simulink library "mylib"  (R2020a)
settings: Solver=VariableStepAuto  StartTime=0.0  StopTime=10.0  RelTol=1e-3
undefined symbols (not defined in the file): d_du_max_pu, dir_to_bus1, dir_to_bus_0L, dir_to_bus_2, dir_to_line1, dir_to_line_0L, dir_to_line_2, du_max_pu, du_ph_max_pu, Fi_0, Fi_T_H, Fi_T_L, Fi_T_M, I0_calc_0L, I0_comp_H, I0_comp_L, I0_comp_M, I0_max_0L, I2_max_2, I_diff1, I_diff2, I_diff3, I_diff4, I_diff5, I_diff_to, I_hight_CT1_G, I_hight_CT2_G, I_low_CT1, I_low_CT2, I_max1, I_max2, I_max3, I_max4, I_max5, I_min_sec_CT1, I_min_sec_CT2, I_unb, Iph_max_0L, Iph_max_2, jmp_in_zone, jmp_in_zone_0L, jmp_in_zone_2, K_dop, max_min1, only_K1_0L, only_K1_2, only_K2_0L, only_K2_2, only_K3_0L, only_K3_2, P_ctl_0, PQ_Fi_ctl_0, Q_ctl_0, S_set_0, set, set1, T_fast, T_I_ctl, T_off, T_on ... (+15)
libraries: $bdroot x184, powerlib_meascontrol x97
(part 8 of 14)

== system mylib/Inverse time-delay/ANSI Inverse time-delay/Сoefficient_6 ==
  A_in : Inport
  B_in : Inport  Port=2
  C_in : Inport  Port=3
  N : Inport  Port=4
  Constant1 : Constant  Value=0.02434
  Constant3 : Constant  Value=2
  Constant6 : Constant  Value=5.64
  Switch : Switch  Criteria=u2 > Threshold
  Switch1 : Switch  Criteria=u2 > Threshold
  Switch2 : Switch  Criteria=u2 > Threshold
  A_out : Outport
  B_out : Outport  Port=2
  C_out : Outport  Port=3
  wires:
  Switch1/1 -> B_out/1
  Constant3/1 -> Switch/1
  Constant6/1 -> Switch1/1
  Switch/1 -> A_out/1
  N/1 -> Switch2/2, Switch/2, Switch1/2
  A_in/1 -> Switch/3
  B_in/1 -> Switch1/3
  C_in/1 -> Switch2/3
  Constant1/1 -> Switch2/1
  Switch2/1 -> C_out/1

== system mylib/Inverse time-delay/ANSI Inverse time-delay/Сoefficient_7 ==
  A_in : Inport
  B_in : Inport  Port=2
  C_in : Inport  Port=3
  N : Inport  Port=4
  Constant1 : Constant  Value=0.21359
  Constant3 : Constant  Value=1.5825
  Constant6 : Constant  Value=0.4797
  Switch : Switch  Criteria=u2 > Threshold
  Switch1 : Switch  Criteria=u2 > Threshold
  Switch2 : Switch  Criteria=u2 > Threshold
  A_out : Outport
  B_out : Outport  Port=2
  C_out : Outport  Port=3
  wires:
  Switch1/1 -> B_out/1
  Constant3/1 -> Switch/1
  Constant6/1 -> Switch1/1
  Switch/1 -> A_out/1
  N/1 -> Switch2/2, Switch/2, Switch1/2
  A_in/1 -> Switch/3
  B_in/1 -> Switch1/3
  C_in/1 -> Switch2/3
  Constant1/1 -> Switch2/1
  Switch2/1 -> C_out/1

== system mylib/Inverse time-delay/ANSI Inverse time-delay/Сoefficient_8 User ==
  A_in : Inport
  B_in : Inport  Port=2
  C_in : Inport  Port=3
  N : Inport  Port=4
  Au : Inport  Port=5
  Bu : Inport  Port=6
  Cu : Inport  Port=7
  Switch : Switch  Criteria=u2 > Threshold
  Switch1 : Switch  Criteria=u2 > Threshold
  Switch2 : Switch  Criteria=u2 > Threshold
  B_out : Outport
  A_out : Outport  Port=2
  C_out : Outport  Port=3
  wires:
  Switch1/1 -> B_out/1
  Au/1 -> Switch/1
  Bu/1 -> Switch1/1
  Switch/1 -> A_out/1
  N/1 -> Switch2/2, Switch/2, Switch1/2
  A_in/1 -> Switch/3
  B_in/1 -> Switch1/3
  C_in/1 -> Switch2/3
  Cu/1 -> Switch2/1
  Switch2/1 -> C_out/1

== system mylib/Inverse time-delay/ANSI Inverse time-delay inductive disk relay/Equation ANSI_idr ==
  B : Inport
  I : Inport  Port=2
  Ip : Inport  Port=3
  A : Inport  Port=4
  C : Inport  Port=5
  D : Inport  Port=6
  Add : Sum  Inputs=+-
  Add1 : Sum
  Constant3 : Constant
  Divide : Product  Inputs=*/
  Divide1 : Product  Inputs=*/
  Divide3 : Product  Inputs=**
  Math Function : Math  Operator=pow  SaturateOnIntegerOverflow=on
  Zero_check : Subsystem
  Zero_check1 : Subsystem
  td : Outport
  wires:
  I/1 -> Divide/1
  B/1 -> Divide1/1
  D/1 -> Divide3/2
  Divide3/1 -> td/1
  Divide/1 -> Math Function/1
  A/1 -> Math Function/2
  Ip/1 -> Zero_check/1(in)
  Zero_check/1(out) -> Divide/2
  Add/1 -> Zero_check1/1(in)
  Zero_check1/1(out) -> Divide1/2
  Constant3/1 -> Add/1
  Divide1/1 -> Add1/1
  Add1/1 -> Divide3/1
  C/1 -> Add1/2
  Math Function/1 -> Add/2

== system mylib/Inverse time-delay/ANSI Inverse time-delay inductive disk relay/Сoefficient_1 ==
  A_in : Inport
  B_in : Inport  Port=2
  C_in : Inport  Port=3
  N : Inport  Port=4
  Constant1 : Constant  Value=0
  Constant3 : Constant  Value=2.0938
  Constant6 : Constant  Value=8.8
  Switch : Switch  Criteria=u2 > Threshold
  Switch1 : Switch  Criteria=u2 > Threshold
  Switch2 : Switch  Criteria=u2 > Threshold
  A_out : Outport
  B_out : Outport  Port=2
  C_out : Outport  Port=3
  wires:
  Switch1/1 -> B_out/1
  Constant3/1 -> Switch/1
  Constant6/1 -> Switch1/1
  Switch/1 -> A_out/1
  N/1 -> Switch2/2, Switch/2, Switch1/2
  A_in/1 -> Switch/3
  B_in/1 -> Switch1/3
  C_in/1 -> Switch2/3
  Constant1/1 -> Switch2/1
  Switch2/1 -> C_out/1

== system mylib/Inverse time-delay/ANSI Inverse time-delay inductive disk relay/Сoefficient_2 ==
  A_in : Inport
  B_in : Inport  Port=2
  C_in : Inport  Port=3
  N : Inport  Port=4
  Constant1 : Constant  Value=0
  Constant3 : Constant  Value=1.2969
  Constant6 : Constant  Value=0.831
  Switch : Switch  Criteria=u2 > Threshold
  Switch1 : Switch  Criteria=u2 > Threshold
  Switch2 : Switch  Criteria=u2 > Threshold
  A_out : Outport
  B_out : Outport  Port=2
  C_out : Outport  Port=3
  wires:
  Switch1/1 -> B_out/1
  Constant3/1 -> Switch/1
  Constant6/1 -> Switch1/1
  Switch/1 -> A_out/1
  N/1 -> Switch2/2, Switch/2, Switch1/2
  A_in/1 -> Switch/3
  B_in/1 -> Switch1/3
  C_in/1 -> Switch2/3
  Constant1/1 -> Switch2/1
  Switch2/1 -> C_out/1

== system mylib/Inverse time-delay/ANSI Inverse time-delay inductive disk relay/Сoefficient_3 ==
  A_in : Inport
  B_in : Inport  Port=2
  C_in : Inport  Port=3
  N : Inport  Port=4
  Constant1 : Constant  Value=0
  Constant3 : Constant
  Constant6 : Constant  Value=12.9
  Switch : Switch  Criteria=u2 > Threshold
  Switch1 : Switch  Criteria=u2 > Threshold
  Switch2 : Switch  Criteria=u2 > Threshold
  A_out : Outport
  B_out : Outport  Port=2
  C_out : Outport  Port=3
  wires:
  Switch1/1 -> B_out/1
  Constant3/1 -> Switch/1
  Constant6/1 -> Switch1/1
  Switch/1 -> A_out/1
  N/1 -> Switch2/2, Switch/2, Switch1/2
  A_in/1 -> Switch/3
  B_in/1 -> Switch1/3
  C_in/1 -> Switch2/3
  Constant1/1 -> Switch2/1
  Switch2/1 -> C_out/1

== system mylib/Inverse time-delay/ANSI Inverse time-delay inductive disk relay/Сoefficient_4 ==
  A_in : Inport
  B_in : Inport  Port=2
  C_in : Inport  Port=3
  N : Inport  Port=4
  Constant1 : Constant  Value=0
  Constant3 : Constant  Value=2
  Constant6 : Constant  Value=0.97
  Switch : Switch  Criteria=u2 > Threshold
  Switch1 : Switch  Criteria=u2 > Threshold
  Switch2 : Switch  Criteria=u2 > Threshold
  A_out : Outport
  B_out : Outport  Port=2
  C_out : Outport  Port=3
  wires:
  Switch1/1 -> B_out/1
  Constant3/1 -> Switch/1
  Constant6/1 -> Switch1/1
  Switch/1 -> A_out/1
  N/1 -> Switch2/2, Switch/2, Switch1/2
  A_in/1 -> Switch/3
  B_in/1 -> Switch1/3
  C_in/1 -> Switch2/3
  Constant1/1 -> Switch2/1
  Switch2/1 -> C_out/1

== system mylib/Inverse time-delay/ANSI Inverse time-delay inductive disk relay/Сoefficient_5 ==
  A_in : Inport
  B_in : Inport  Port=2
  C_in : Inport  Port=3
  N : Inport  Port=4
  Constant1 : Constant  Value=0
  Constant3 : Constant  Value=2
  Constant6 : Constant  Value=4.32
  Switch : Switch  Criteria=u2 > Threshold
  Switch1 : Switch  Criteria=u2 > Threshold
  Switch2 : Switch  Criteria=u2 > Threshold
  A_out : Outport
  B_out : Outport  Port=2
  C_out : Outport  Port=3
  wires:
  Switch1/1 -> B_out/1
  Constant3/1 -> Switch/1
  Constant6/1 -> Switch1/1
  Switch/1 -> A_out/1
  N/1 -> Switch2/2, Switch/2, Switch1/2
  A_in/1 -> Switch/3
  B_in/1 -> Switch1/3
  C_in/1 -> Switch2/3
  Constant1/1 -> Switch2/1
  Switch2/1 -> C_out/1

== system mylib/Inverse time-delay/ANSI Inverse time-delay inductive disk relay/Сoefficient_6 ==
  A_in : Inport
  B_in : Inport  Port=2
  C_in : Inport  Port=3
  N : Inport  Port=4
  Constant1 : Constant  Value=0
  Constant3 : Constant  Value=2
  Constant6 : Constant  Value=5.82
  Switch : Switch  Criteria=u2 > Threshold
  Switch1 : Switch  Criteria=u2 > Threshold
  Switch2 : Switch  Criteria=u2 > Threshold
  A_out : Outport
  B_out : Outport  Port=2
  C_out : Outport  Port=3
  wires:
  Switch1/1 -> B_out/1
  Constant3/1 -> Switch/1
  Constant6/1 -> Switch1/1
  Switch/1 -> A_out/1
  N/1 -> Switch2/2, Switch/2, Switch1/2
  A_in/1 -> Switch/3
  B_in/1 -> Switch1/3
  C_in/1 -> Switch2/3
  Constant1/1 -> Switch2/1
  Switch2/1 -> C_out/1

== system mylib/Inverse time-delay/ANSI Inverse time-delay inductive disk relay/Сoefficient_7 ==
  A_in : Inport
  B_in : Inport  Port=2
  C_in : Inport  Port=3
  N : Inport  Port=4
  Constant1 : Constant  Value=0.21359
  Constant3 : Constant  Value=1.5625
  Constant6 : Constant  Value=1.0394
  Switch : Switch  Criteria=u2 > Threshold
  Switch1 : Switch  Criteria=u2 > Threshold
  Switch2 : Switch  Criteria=u2 > Threshold
  A_out : Outport
  B_out : Outport  Port=2
  C_out : Outport  Port=3
  wires:
  Switch1/1 -> B_out/1
  Constant3/1 -> Switch/1
  Constant6/1 -> Switch1/1
  Switch/1 -> A_out/1
  N/1 -> Switch2/2, Switch/2, Switch1/2
  A_in/1 -> Switch/3
  B_in/1 -> Switch1/3
  C_in/1 -> Switch2/3
  Constant1/1 -> Switch2/1
  Switch2/1 -> C_out/1

== system mylib/Inverse time-delay/ANSI Inverse time-delay inductive disk relay/Сoefficient_8 User ==
  A_in : Inport
  B_in : Inport  Port=2
  C_in : Inport  Port=3
  N : Inport  Port=4
  Au : Inport  Port=5
  Bu : Inport  Port=6
  Cu : Inport  Port=7
  Switch : Switch  Criteria=u2 > Threshold
  Switch1 : Switch  Criteria=u2 > Threshold
  Switch2 : Switch  Criteria=u2 > Threshold
  B_out : Outport
  A_out : Outport  Port=2
  C_out : Outport  Port=3
  wires:
  Switch1/1 -> B_out/1
  Au/1 -> Switch/1
  Bu/1 -> Switch1/1
  Switch/1 -> A_out/1
  N/1 -> Switch2/2, Switch/2, Switch1/2
  A_in/1 -> Switch/3
  B_in/1 -> Switch1/3
  C_in/1 -> Switch2/3
  Cu/1 -> Switch2/1
  Switch2/1 -> C_out/1

== system mylib/Inverse time-delay/IEC Inverse time-delay/Equation IEC ==
  k : Inport
  I : Inport  Port=2
  a : Inport  Port=3
  Ip : Inport  Port=4
  Tb : Inport  Port=5
  Add : Sum  Inputs=+-
  Constant18 : Constant  Value=20
  Constant3 : Constant
  Divide : Product  Inputs=*/
  Divide1 : Product  Inputs=*/
  Divide2 : Product  Inputs=*/
  Divide3 : Product  Inputs=**
  Math Function : Math  Operator=pow  SaturateOnIntegerOverflow=on
  Relational Operator : RelationalOperator  OutDataTypeStr=boolean  RndMeth=Simplest
  Switch : Switch  Criteria=u2 > Threshold
  Zero_check : Subsystem
  Zero_check1 : Subsystem
  td : Outport
  wires:
  I/1 -> Divide/1, Divide2/1
  Math Function/1 -> Add/1
  Constant3/1 -> Add/2
  k/1 -> Divide1/1
  Divide1/1 -> Divide3/1
  Tb/1 -> Divide3/2
  Divide3/1 -> td/1
  a/1 -> Math Function/2
  Ip/1 -> Zero_check/1(in)
  Zero_check/1(out) -> Divide2/2, Divide/2
  Add/1 -> Zero_check1/1(in)
  Zero_check1/1(out) -> Divide1/2
  Divide2/1 -> Relational Operator/1
  Constant18/1 -> Switch/1, Relational Operator/2
  Relational Operator/1 -> Switch/2
  Divide/1 -> Switch/3
  Switch/1 -> Math Function/1

== system mylib/Inverse time-delay/IEC Inverse time-delay/Сoefficient_1 ==
  k_in : Inport
  a_in : Inport  Port=2
  N : Inport  Port=3
  Constant3 : Constant  Value=0.14
  Constant6 : Constant  Value=0.02
  Switch : Switch  Criteria=u2 > Threshold
  Switch1 : Switch  Criteria=u2 > Threshold
  k_out : Outport
  a_out : Outport  Port=2
  wires:
  Switch1/1 -> a_out/1
  Constant3/1 -> Switch/1
  Constant6/1 -> Switch1/1
  Switch/1 -> k_out/1
  N/1 -> Switch/2, Switch1/2
  k_in/1 -> Switch/3
  a_in/1 -> Switch1/3

== system mylib/Inverse time-delay/IEC Inverse time-delay/Сoefficient_2 ==
  k_in : Inport
  a_in : Inport  Port=2
  N : Inport  Port=3
  Constant3 : Constant  Value=13.5
  Constant6 : Constant
  Switch : Switch  Criteria=u2 > Threshold
  Switch1 : Switch  Criteria=u2 > Threshold
  k_out : Outport
  a_out : Outport  Port=2
  wires:
  Switch1/1 -> a_out/1
  Constant3/1 -> Switch/1
  Constant6/1 -> Switch1/1
  Switch/1 -> k_out/1
  N/1 -> Switch/2, Switch1/2
  k_in/1 -> Switch/3
  a_in/1 -> Switch1/3

== system mylib/Inverse time-delay/IEC Inverse time-delay/Сoefficient_3 ==
  k_in : Inport
  a_in : Inport  Port=2
  N : Inport  Port=3
  Constant3 : Constant  Value=120
  Constant6 : Constant
  Switch : Switch  Criteria=u2 > Threshold
  Switch1 : Switch  Criteria=u2 > Threshold
  k_out : Outport
  a_out : Outport  Port=2
  wires:
  Switch1/1 -> a_out/1
  Constant3/1 -> Switch/1
  Constant6/1 -> Switch1/1
  Switch/1 -> k_out/1
  N/1 -> Switch/2, Switch1/2
  k_in/1 -> Switch/3
  a_in/1 -> Switch1/3

== system mylib/Inverse time-delay/IEC Inverse time-delay/Сoefficient_4 ==
  k_in : Inport
  a_in : Inport  Port=2
  N : Inport  Port=3
  Constant3 : Constant  Value=80
  Constant6 : Constant  Value=2
  Switch : Switch  Criteria=u2 > Threshold
  Switch1 : Switch  Criteria=u2 > Threshold
  k_out : Outport
  a_out : Outport  Port=2
  wires:
  Switch1/1 -> a_out/1
  Constant3/1 -> Switch/1
  Constant6/1 -> Switch1/1
  Switch/1 -> k_out/1
  N/1 -> Switch/2, Switch1/2
  k_in/1 -> Switch/3
  a_in/1 -> Switch1/3

== system mylib/Inverse time-delay/IEC Inverse time-delay/Сoefficient_5 User ==
  k : Inport
  a : Inport  Port=2
  N : Inport  Port=3
  k_u : Inport  Port=4
  a_u : Inport  Port=5
  Switch : Switch  Criteria=u2 > Threshold
  Switch1 : Switch  Criteria=u2 > Threshold
  k_out : Outport
  a_out : Outport  Port=2
  wires:
  Switch1/1 -> a_out/1
  k_u/1 -> Switch/1
  a_u/1 -> Switch1/1
  Switch/1 -> k_out/1
  N/1 -> Switch/2, Switch1/2
  k/1 -> Switch/3
  a/1 -> Switch1/3

== system mylib/Inverse time-delay/IEC Inverse time-delay inductive disk relay/Equation IEC_idr ==
  k : Inport
  I : Inport  Port=2
  a : Inport  Port=3
  Ip : Inport  Port=4
  Tb : Inport  Port=5
  Add : Sum  Inputs=+-
  Constant3 : Constant
  Divide : Product  Inputs=*/
  Divide1 : Product  Inputs=*/
  Divide3 : Product  Inputs=**
  Math Function : Math  Operator=pow  SaturateOnIntegerOverflow=on
  Zero_check : Subsystem
  Zero_check1 : Subsystem
  td : Outport
  wires:
  I/1 -> Divide/1
  k/1 -> Divide1/1
  Divide1/1 -> Divide3/1
  Tb/1 -> Divide3/2
  Divide3/1 -> td/1
  Divide/1 -> Math Function/1
  a/1 -> Math Function/2
  Ip/1 -> Zero_check/1(in)
  Zero_check/1(out) -> Divide/2
  Add/1 -> Zero_check1/1(in)
  Zero_check1/1(out) -> Divide1/2
  Math Function/1 -> Add/2
  Constant3/1 -> Add/1

== system mylib/Inverse time-delay/IEC Inverse time-delay inductive disk relay/Сoefficient_1 ==
  k_in : Inport
  a_in : Inport  Port=2
  N : Inport  Port=3
  Constant3 : Constant  Value=9.7
  Constant6 : Constant  Value=2
  Switch : Switch  Criteria=u2 > Threshold
  Switch1 : Switch  Criteria=u2 > Threshold
  k_out : Outport
  a_out : Outport  Port=2
  wires:
  Switch1/1 -> a_out/1
  Constant3/1 -> Switch/1
  Constant6/1 -> Switch1/1
  Switch/1 -> k_out/1
  N/1 -> Switch/2, Switch1/2
  k_in/1 -> Switch/3
  a_in/1 -> Switch1/3

== system mylib/Inverse time-delay/IEC Inverse time-delay inductive disk relay/Сoefficient_2 ==
  k_in : Inport
  a_in : Inport  Port=2
  N : Inport  Port=3
  Constant3 : Constant  Value=43.2
  Constant6 : Constant  Value=2
  Switch : Switch  Criteria=u2 > Threshold
  Switch1 : Switch  Criteria=u2 > Threshold
  k_out : Outport
  a_out : Outport  Port=2
  wires:
  Switch1/1 -> a_out/1
  Constant3/1 -> Switch/1
  Constant6/1 -> Switch1/1
  Switch/1 -> k_out/1
  N/1 -> Switch/2, Switch1/2
  k_in/1 -> Switch/3
  a_in/1 -> Switch1/3

== system mylib/Inverse time-delay/IEC Inverse time-delay inductive disk relay/Сoefficient_3 ==
  k_in : Inport
  a_in : Inport  Port=2
  N : Inport  Port=3
  Constant3 : Constant  Value=58.2
  Constant6 : Constant  Value=2
  Switch : Switch  Criteria=u2 > Threshold
  Switch1 : Switch  Criteria=u2 > Threshold
  k_out : Outport
  a_out : Outport  Port=2
  wires:
  Switch1/1 -> a_out/1
  Constant3/1 -> Switch/1
  Constant6/1 -> Switch1/1
  Switch/1 -> k_out/1
  N/1 -> Switch/2, Switch1/2
  k_in/1 -> Switch/3
  a_in/1 -> Switch1/3

== system mylib/Inverse time-delay/IEC Inverse time-delay inductive disk relay/Сoefficient_4 ==
  k_in : Inport
  a_in : Inport  Port=2
  N : Inport  Port=3
  Constant3 : Constant  Value=80
  Constant6 : Constant  Value=2
  Switch : Switch  Criteria=u2 > Threshold
  Switch1 : Switch  Criteria=u2 > Threshold
  k_out : Outport
  a_out : Outport  Port=2
  wires:
  Switch1/1 -> a_out/1
  Constant3/1 -> Switch/1
  Constant6/1 -> Switch1/1
  Switch/1 -> k_out/1
  N/1 -> Switch/2, Switch1/2
  k_in/1 -> Switch/3
  a_in/1 -> Switch1/3

== system mylib/Inverse time-delay/IEC Inverse time-delay inductive disk relay/Сoefficient_5 User ==
  k : Inport
  a : Inport  Port=2
  N : Inport  Port=3
  k_u : Inport  Port=4
  a_u : Inport  Port=5
  Switch : Switch  Criteria=u2 > Threshold
  Switch1 : Switch  Criteria=u2 > Threshold
  k_out : Outport
  a_out : Outport  Port=2
  wires:
  Switch1/1 -> a_out/1
  k_u/1 -> Switch/1
  a_u/1 -> Switch1/1
  Switch/1 -> k_out/1
  N/1 -> Switch/2, Switch1/2
  k/1 -> Switch/3
  a/1 -> Switch1/3

== system mylib/st_inverse/Inverse time-delay/ANSI Inverse time-delay ==
  I : Inport
  ANSI_N : Inport  Port=2
  Au_ANSI : Inport  Port=3
  Bu_ANSI : Inport  Port=4
  Cu_ANSI : Inport  Port=5
  Ip : Inport  Port=6
  D : Inport  Port=7
  Constant1 : Constant  Value=6
  Constant2 : Constant  Value=7
  Constant20 : Constant
  Constant21 : Constant  Value=2
  Constant22 : Constant  Value=3
  Constant23 : Constant  Value=4
  Constant25 : Constant  Value=5
  Constant3 : Constant  Value=0
  Constant4 : Constant  Value=8
  Equation ANSI : Subsystem
  Relational Operator{,1..7} (8 alike) : RelationalOperator  Operator===  OutDataTypeStr=boolean  RndMeth=Simplest
  Сoefficient_1 : Subsystem
  Сoefficient_2 : Subsystem
  Сoefficient_3 : Subsystem
  Сoefficient_4 : Subsystem
  Сoefficient_5 : Subsystem
  Сoefficient_6 : Subsystem
  Сoefficient_7 : Subsystem
  Сoefficient_8 User : Subsystem
  td : Outport
  wires:
  Relational Operator/1 -> Сoefficient_1/4(N)
  Constant25/1 -> Relational Operator5/2
  Constant22/1 -> Relational Operator2/2
  Constant3/1 -> Сoefficient_1/3(C_in), Сoefficient_1/2(B_in), Сoefficient_1/1(A_in)
  ANSI_N/1 -> Relational Operator1/1, Relational Operator2/1, Relational Operator7/1, Relational Operator6/1, Relational Operator4/1, Relational Operator5/1, Relational Operator3/1, Relational Operator/1
  Constant23/1 -> Relational Operator3/2
  D/1 -> Equation ANSI/6(D)
  Constant21/1 -> Relational Operator1/2
  Constant20/1 -> Relational Operator/2
  I/1 -> Equation ANSI/2(I)
  Ip/1 -> Equation ANSI/3(Ip)
  Equation ANSI/1(td) -> td/1
  Сoefficient_1/1(A_out) -> Сoefficient_2/1(A_in)
  Сoefficient_1/2(B_out) -> Сoefficient_2/2(B_in)
  Сoefficient_1/3(C_out) -> Сoefficient_2/3(C_in)
  Relational Operator1/1 -> Сoefficient_2/4(N)
  Сoefficient_2/1(A_out) -> Сoefficient_3/1(A_in)
  Сoefficient_2/2(B_out) -> Сoefficient_3/2(B_in)
  Сoefficient_2/3(C_out) -> Сoefficient_3/3(C_in)
  Relational Operator2/1 -> Сoefficient_3/4(N)
  Сoefficient_3/1(A_out) -> Сoefficient_4/1(A_in)
  Сoefficient_3/2(B_out) -> Сoefficient_4/2(B_in)
  Сoefficient_3/3(C_out) -> Сoefficient_4/3(C_in)
  Relational Operator3/1 -> Сoefficient_4/4(N)
  Сoefficient_4/1(A_out) -> Сoefficient_5/1(A_in)
  Сoefficient_4/2(B_out) -> Сoefficient_5/2(B_in)
  Сoefficient_4/3(C_out) -> Сoefficient_5/3(C_in)
  Relational Operator5/1 -> Сoefficient_5/4(N)
  Сoefficient_8 User/1(B_out) -> Equation ANSI/1(B)
  Сoefficient_8 User/2(A_out) -> Equation ANSI/4(A)
  Сoefficient_8 User/3(C_out) -> Equation ANSI/5(C)
  Au_ANSI/1 -> Сoefficient_8 User/5(Au)
  Bu_ANSI/1 -> Сoefficient_8 User/6(Bu)
  Cu_ANSI/1 -> Сoefficient_8 User/7(Cu)
  Сoefficient_5/1(A_out) -> Сoefficient_6/1(A_in)
  Сoefficient_5/2(B_out) -> Сoefficient_6/2(B_in)
  Сoefficient_5/3(C_out) -> Сoefficient_6/3(C_in)
  Constant4/1 -> Relational Operator7/2
  Constant2/1 -> Relational Operator6/2
  Constant1/1 -> Relational Operator4/2
  Relational Operator7/1 -> Сoefficient_8 User/4(N)
  Сoefficient_6/1(A_out) -> Сoefficient_7/1(A_in)
  Сoefficient_6/2(B_out) -> Сoefficient_7/2(B_in)
  Сoefficient_6/3(C_out) -> Сoefficient_7/3(C_in)
  Relational Operator6/1 -> Сoefficient_7/4(N)
  Relational Operator4/1 -> Сoefficient_6/4(N)
  Сoefficient_7/3(C_out) -> Сoefficient_8 User/3(C_in)
  Сoefficient_7/2(B_out) -> Сoefficient_8 User/2(B_in)
  Сoefficient_7/1(A_out) -> Сoefficient_8 User/1(A_in)

== system mylib/st_inverse/Inverse time-delay/ANSI Inverse time-delay inductive disk relay ==
  I : Inport
  ANSI_N_idr : Inport  Port=2
  Au_ANSI_idr : Inport  Port=3
  Bu_ANSI_idr : Inport  Port=4
  Cu_ANSI_idr : Inport  Port=5
  Ip : Inport  Port=6
  D : Inport  Port=7
  Constant1 : Constant  Value=6
  Constant2 : Constant  Value=7
  Constant20 : Constant
  Constant21 : Constant  Value=2
  Constant22 : Constant  Value=3
  Constant23 : Constant  Value=4
  Constant25 : Constant  Value=5
  Constant3 : Constant  Value=0
  Constant4 : Constant  Value=8
  Equation ANSI_idr : Subsystem
  Relational Operator{,1..7} (8 alike) : RelationalOperator  Operator===  OutDataTypeStr=boolean  RndMeth=Simplest
  Сoefficient_1 : Subsystem
  Сoefficient_2 : Subsystem
  Сoefficient_3 : Subsystem
  Сoefficient_4 : Subsystem
  Сoefficient_5 : Subsystem
  Сoefficient_6 : Subsystem
  Сoefficient_7 : Subsystem
  Сoefficient_8 User : Subsystem
  td : Outport
  wires:
  Relational Operator/1 -> Сoefficient_1/4(N)
  Constant25/1 -> Relational Operator5/2
  Constant22/1 -> Relational Operator2/2
  Constant3/1 -> Сoefficient_1/3(C_in), Сoefficient_1/2(B_in), Сoefficient_1/1(A_in)
  ANSI_N_idr/1 -> Relational Operator1/1, Relational Operator2/1, Relational Operator7/1, Relational Operator6/1, Relational Operator4/1, Relational Operator5/1, Relational Operator3/1, Relational Operator/1
  Constant23/1 -> Relational Operator3/2
  D/1 -> Equation ANSI_idr/6(D)
  Constant21/1 -> Relational Operator1/2
  Constant20/1 -> Relational Operator/2
  I/1 -> Equation ANSI_idr/2(I)
  Ip/1 -> Equation ANSI_idr/3(Ip)
  Equation ANSI_idr/1(td) -> td/1
  Сoefficient_1/1(A_out) -> Сoefficient_2/1(A_in)
  Сoefficient_1/2(B_out) -> Сoefficient_2/2(B_in)
  Сoefficient_1/3(C_out) -> Сoefficient_2/3(C_in)
  Relational Operator1/1 -> Сoefficient_2/4(N)
  Сoefficient_2/1(A_out) -> Сoefficient_3/1(A_in)
  Сoefficient_2/2(B_out) -> Сoefficient_3/2(B_in)
  Сoefficient_2/3(C_out) -> Сoefficient_3/3(C_in)
  Relational Operator2/1 -> Сoefficient_3/4(N)
  Сoefficient_3/1(A_out) -> Сoefficient_4/1(A_in)
  Сoefficient_3/2(B_out) -> Сoefficient_4/2(B_in)
  Сoefficient_3/3(C_out) -> Сoefficient_4/3(C_in)
  Relational Operator3/1 -> Сoefficient_4/4(N)
  Сoefficient_4/1(A_out) -> Сoefficient_5/1(A_in)
  Сoefficient_4/2(B_out) -> Сoefficient_5/2(B_in)
  Сoefficient_4/3(C_out) -> Сoefficient_5/3(C_in)
  Relational Operator5/1 -> Сoefficient_5/4(N)
  Сoefficient_8 User/1(B_out) -> Equation ANSI_idr/1(B)
  Сoefficient_8 User/2(A_out) -> Equation ANSI_idr/4(A)
  Сoefficient_8 User/3(C_out) -> Equation ANSI_idr/5(C)
  Au_ANSI_idr/1 -> Сoefficient_8 User/5(Au)
  Bu_ANSI_idr/1 -> Сoefficient_8 User/6(Bu)
  Cu_ANSI_idr/1 -> Сoefficient_8 User/7(Cu)
  Сoefficient_5/1(A_out) -> Сoefficient_6/1(A_in)
  Сoefficient_5/2(B_out) -> Сoefficient_6/2(B_in)
  Сoefficient_5/3(C_out) -> Сoefficient_6/3(C_in)
  Constant4/1 -> Relational Operator7/2
  Constant2/1 -> Relational Operator6/2
  Constant1/1 -> Relational Operator4/2
  Relational Operator7/1 -> Сoefficient_8 User/4(N)
  Сoefficient_6/1(A_out) -> Сoefficient_7/1(A_in)
  Сoefficient_6/2(B_out) -> Сoefficient_7/2(B_in)
  Сoefficient_6/3(C_out) -> Сoefficient_7/3(C_in)
  Relational Operator6/1 -> Сoefficient_7/4(N)
  Relational Operator4/1 -> Сoefficient_6/4(N)
  Сoefficient_7/3(C_out) -> Сoefficient_8 User/3(C_in)
  Сoefficient_7/2(B_out) -> Сoefficient_8 User/2(B_in)
  Сoefficient_7/1(A_out) -> Сoefficient_8 User/1(A_in)

== system mylib/st_inverse/Inverse time-delay/IEC Inverse time-delay ==
  I : Inport
  IEC_N : Inport  Port=2
  ku_IEC : Inport  Port=3
  au_IEC : Inport  Port=4
  Ip : Inport  Port=5
  Tb : Inport  Port=6
  Constant20 : Constant
  Constant21 : Constant  Value=2
  Constant22 : Constant  Value=3
  Constant23 : Constant  Value=4
  Constant25 : Constant  Value=5
  Constant3 : Constant  Value=0
  Equation IEC : Subsystem
  Relational Operator{,1..3,5} (5 alike) : RelationalOperator  Operator===  OutDataTypeStr=boolean  RndMeth=Simplest
  Сoefficient_1 : Subsystem
  Сoefficient_2 : Subsystem
  Сoefficient_3 : Subsystem
  Сoefficient_4 : Subsystem
  Сoefficient_5 User : Subsystem
  td : Outport
  wires:
  Сoefficient_5 User/1(k_out) -> Equation IEC/1(k)
  Сoefficient_1/1(k_out) -> Сoefficient_2/1(k_in)
  Relational Operator/1 -> Сoefficient_1/3(N)
  Relational Operator3/1 -> Сoefficient_4/3(N)
  Constant25/1 -> Relational Operator5/2
  Constant22/1 -> Relational Operator2/2
  Constant3/1 -> Сoefficient_1/2(a_in), Сoefficient_1/1(k_in)
  Relational Operator2/1 -> Сoefficient_3/3(N)
  IEC_N/1 -> Relational Operator1/1, Relational Operator2/1, Relational Operator5/1, Relational Operator3/1, Relational Operator/1
  Constant23/1 -> Relational Operator3/2
  Сoefficient_5 User/2(a_out) -> Equation IEC/3(a)
  Tb/1 -> Equation IEC/5(Tb)
  Relational Operator1/1 -> Сoefficient_2/3(N)
  Constant21/1 -> Relational Operator1/2
  Constant20/1 -> Relational Operator/2
  I/1 -> Equation IEC/2(I)
  Сoefficient_1/2(a_out) -> Сoefficient_2/2(a_in)
  Relational Operator5/1 -> Сoefficient_5 User/3(N)
  Ip/1 -> Equation IEC/4(Ip)
  Equation IEC/1(td) -> td/1
  ku_IEC/1 -> Сoefficient_5 User/4(k_u)
  au_IEC/1 -> Сoefficient_5 User/5(a_u)
  Сoefficient_2/2(a_out) -> Сoefficient_3/2(a_in)
  Сoefficient_2/1(k_out) -> Сoefficient_3/1(k_in)
  Сoefficient_3/1(k_out) -> Сoefficient_4/1(k_in)
  Сoefficient_3/2(a_out) -> Сoefficient_4/2(a_in)
  Сoefficient_4/1(k_out) -> Сoefficient_5 User/1(k)
  Сoefficient_4/2(a_out) -> Сoefficient_5 User/2(a)

== system mylib/st_inverse/Inverse time-delay/IEC Inverse time-delay inductive disk relay ==
  I : Inport
  IEC_N_idr : Inport  Port=2
  ku_IEC_idr : Inport  Port=3
  au_IEC_idr : Inport  Port=4
  Ip : Inport  Port=5
  Tb : Inport  Port=6
  Constant20 : Constant
  Constant21 : Constant  Value=2
  Constant22 : Constant  Value=3
  Constant23 : Constant  Value=4
  Constant25 : Constant  Value=5
  Constant3 : Constant  Value=0
  Equation IEC_idr : Subsystem
  Relational Operator{,1..3,5} (5 alike) : RelationalOperator  Operator===  OutDataTypeStr=boolean  RndMeth=Simplest
  Сoefficient_1 : Subsystem
  Сoefficient_2 : Subsystem
  Сoefficient_3 : Subsystem
  Сoefficient_4 : Subsystem
  Сoefficient_5 User : Subsystem
  td : Outport
  wires:
  Сoefficient_5 User/1(k_out) -> Equation IEC_idr/1(k)
  Сoefficient_1/1(k_out) -> Сoefficient_2/1(k_in)
  Relational Operator/1 -> Сoefficient_1/3(N)
  Relational Operator3/1 -> Сoefficient_4/3(N)
  Constant25/1 -> Relational Operator5/2
  Constant22/1 -> Relational Operator2/2
  Constant3/1 -> Сoefficient_1/2(a_in), Сoefficient_1/1(k_in)
  Сoefficient_4/2(a_out) -> Сoefficient_5 User/2(a)
  Relational Operator2/1 -> Сoefficient_3/3(N)
  IEC_N_idr/1 -> Relational Operator1/1, Relational Operator2/1, Relational Operator5/1, Relational Operator3/1, Relational Operator/1
  Constant23/1 -> Relational Operator3/2
  Сoefficient_4/1(k_out) -> Сoefficient_5 User/1(k)
  Сoefficient_5 User/2(a_out) -> Equation IEC_idr/3(a)
  Tb/1 -> Equation IEC_idr/5(Tb)
  Relational Operator1/1 -> Сoefficient_2/3(N)
  Constant21/1 -> Relational Operator1/2
  Constant20/1 -> Relational Operator/2
  I/1 -> Equation IEC_idr/2(I)
  Сoefficient_1/2(a_out) -> Сoefficient_2/2(a_in)
  Relational Operator5/1 -> Сoefficient_5 User/3(N)
  Ip/1 -> Equation IEC_idr/4(Ip)
  Equation IEC_idr/1(td) -> td/1
  ku_IEC_idr/1 -> Сoefficient_5 User/4(k_u)
  au_IEC_idr/1 -> Сoefficient_5 User/5(a_u)
  Сoefficient_2/2(a_out) -> Сoefficient_3/2(a_in)
  Сoefficient_2/1(k_out) -> Сoefficient_3/1(k_in)
  Сoefficient_3/1(k_out) -> Сoefficient_4/1(k_in)
  Сoefficient_3/2(a_out) -> Сoefficient_4/2(a_in)

== system mylib/tzop_st_v1/230_st18_ph/Subsystem ==
  T_fast_time : Inport
  T_fast_zero : Inport  Port=2
  "In1 " : Inport  Port=3
  "In2 " : Inport  Port=4
  "In3 " : Inport  Port=5
  {1..5,7} (6 alike) : Switch  Criteria=u2 > Threshold
  T1 : powerlib_meascontrol/Logic/On Delay  DelayType=On delay  delay=T_st  ic=1  Ts=0
  T2 : powerlib_meascontrol/Logic/On Delay  DelayType=On delay  delay=T_st  ic=1  Ts=0
  T3 : powerlib_meascontrol/Logic/On Delay  DelayType=On delay  delay=T_st  ic=1  Ts=0
  T4 : powerlib_meascontrol/Logic/On Delay  DelayType=On delay  delay=T_fast  ic=1  Ts=0
  T5 : powerlib_meascontrol/Logic/On Delay  DelayType=On delay  delay=T_fast  ic=1  Ts=0
  T6 : powerlib_meascontrol/Logic/On Delay  DelayType=On delay  delay=T_fast  ic=1  Ts=0
  T7 : powerlib_meascontrol/Logic/On Delay  DelayType=Off delay  delay=T_fast  ic=1  Ts=0
  Out1 : Outport
  Out2 : Outport  Port=2
  Out3 : Outport  Port=3
  wires:
  4/1 -> Out3/1
  3/1 -> Out2/1
  5/1 -> Out1/1
  2/1 -> 4/3
  1/1 -> 3/3
  7/1 -> 5/3
  T_fast_zero/1 -> 4/2, 3/2, 5/2
  T2/1 -> 2/3
  T1/1 -> 1/3
  T3/1 -> 7/3
  T6/1 -> 7/1
  T5/1 -> 1/1
  T4/1 -> 2/1
  T_fast_time/1 -> T7/1
  T7/1 -> 7/2, 1/2, 2/2
  "In1 "/1 -> T6/1, T3/1, 5/1
  "In2 "/1 -> T1/1, T5/1, 3/1
  "In3 "/1 -> 4/1, T2/1, T4/1

== system mylib/tzop_st_v1/230_st18_ph/in_1 ==
  jmp_in_zone : Inport
  in : Inport  Port=2
  jmp : Inport  Port=3
  1 : Switch  Criteria=u2 > Threshold
  10 : Logic  AllPortsSameDT=off  OutDataTypeStr=boolean
  11 : Logic  Operator=NOT  AllPortsSameDT=off  OutDataTypeStr=boolean
  12 : Memory
  3 : Logic  AllPortsSameDT=off  OutDataTypeStr=boolean
  RS : $bdroot/RS  SystemSampleTime=-1  Latency=0  AutoFrameSizeCalculation=off
  R_TRIG : $bdroot/R_TRIG  SystemSampleTime=-1  Latency=0  AutoFrameSizeCalculation=off
  T1 : powerlib_meascontrol/Logic/On Delay  DelayType=Off delay  delay=T_reset  ic=1  Ts=0
  T2 : powerlib_meascontrol/Logic/On Delay  DelayType=On delay  delay=T_reset  ic=1  Ts=0
  Y : Outport
  wires:
  3/1 -> RS/1
  T2/1 -> RS/2
  12/1 -> 10/1
  jmp/1 -> T1/1
  1/1 -> 3/1
  T1/1 -> 3/2
  10/1 -> T2/1
  11/1 -> 10/2
  jmp_in_zone/1 -> 1/2
  R_TRIG/1 -> 1/1
  in/1 -> 1/3, R_TRIG/1, 11/1
  RS/1 -> Y/1, 12/1

== system mylib/tzop_st_v1/230_st18_ph/in_2 ==
  jmp_in_zone : Inport
  in : Inport  Port=2
  jmp : Inport  Port=3
  1 : Switch  Criteria=u2 > Threshold
  10 : Logic  AllPortsSameDT=off  OutDataTypeStr=boolean
  11 : Logic  Operator=NOT  AllPortsSameDT=off  OutDataTypeStr=boolean
  12 : Memory
  3 : Logic  AllPortsSameDT=off  OutDataTypeStr=boolean
  RS : $bdroot/RS  SystemSampleTime=-1  Latency=0  AutoFrameSizeCalculation=off
  R_TRIG : $bdroot/R_TRIG  SystemSampleTime=-1  Latency=0  AutoFrameSizeCalculation=off
  T1 : powerlib_meascontrol/Logic/On Delay  DelayType=Off delay  delay=T_reset  ic=1  Ts=0
  T2 : powerlib_meascontrol/Logic/On Delay  DelayType=On delay  delay=T_reset  ic=1  Ts=0
  Y : Outport
  wires:
  3/1 -> RS/1
  T2/1 -> RS/2
  12/1 -> 10/1
  jmp/1 -> T1/1
  1/1 -> 3/1
  T1/1 -> 3/2
  10/1 -> T2/1
  11/1 -> 10/2
  jmp_in_zone/1 -> 1/2
  R_TRIG/1 -> 1/1
  in/1 -> 1/3, R_TRIG/1, 11/1
  RS/1 -> Y/1, 12/1

== system mylib/tzop_st_v1/230_st18_ph/in_3 ==
  jmp_in_zone : Inport
  in : Inport  Port=2
  jmp : Inport  Port=3
  1 : Switch  Criteria=u2 > Threshold
  10 : Logic  AllPortsSameDT=off  OutDataTypeStr=boolean
  11 : Logic  Operator=NOT  AllPortsSameDT=off  OutDataTypeStr=boolean
  12 : Memory
  3 : Logic  AllPortsSameDT=off  OutDataTypeStr=boolean
  RS : $bdroot/RS  SystemSampleTime=-1  Latency=0  AutoFrameSizeCalculation=off
  R_TRIG : $bdroot/R_TRIG  SystemSampleTime=-1  Latency=0  AutoFrameSizeCalculation=off
  T1 : powerlib_meascontrol/Logic/On Delay  DelayType=Off delay  delay=T_reset  ic=1  Ts=0
  T2 : powerlib_meascontrol/Logic/On Delay  DelayType=On delay  delay=T_reset  ic=1  Ts=0
  Y : Outport
  wires:
  3/1 -> RS/1
  T2/1 -> RS/2
  12/1 -> 10/1
  jmp/1 -> T1/1
  1/1 -> 3/1
  T1/1 -> 3/2
  10/1 -> T2/1
  11/1 -> 10/2
  jmp_in_zone/1 -> 1/2
  R_TRIG/1 -> 1/1
  in/1 -> 1/3, R_TRIG/1, 11/1
  RS/1 -> Y/1, 12/1

== system mylib/tzop_st_v1/230_st18_ph/k_type ==
  In_a : Inport
  In_b : Inport  Port=2
  In_ c : Inport  Port=3
  only_K1 : Inport  Port=4
  only_K2 : Inport  Port=5
  only_K3 : Inport  Port=6
  1 : Switch  Criteria=u2 > Threshold
  Logical Operator{1,12,18..27} (12 alike) : Logic  Operator=NOT  AllPortsSameDT=off  OutDataTypeStr=boolean
  Logical Operator10 : Logic  AllPortsSameDT=off  OutDataTypeStr=boolean
  Logical Operator{2..4,7..8,11,14,17} (8 alike) : Logic  Inputs=3  AllPortsSameDT=off  OutDataTypeStr=boolean
  Logical Operator{5..6,13,16} (4 alike) : Logic  Operator=OR  Inputs=3  AllPortsSameDT=off  OutDataTypeStr=boolean
  Logical Operator15 : Logic  AllPortsSameDT=off  OutDataTypeStr=boolean
  Logical Operator9 : Logic  AllPortsSameDT=off  OutDataTypeStr=boolean
  out : Outport
  wires:
  In_ c/1 -> Logical Operator14/3, Logical Operator16/3, Logical Operator21/1, Logical Operator7/3, Logical Operator4/3, Logical Operator3/3, Logical Operator25/1, Logical Operator1/1
  Logical Operator16/1 -> 1/1
  Logical Operator13/1 -> 1/3
  1/1 -> out/1
  Logical Operator17/1 -> 1/2
  only_K3/1 -> Logical Operator20/1, Logical Operator15/1
  only_K2/1 -> Logical Operator10/1, Logical Operator18/1
  only_K1/1 -> Logical Operator9/1, Logical Operator19/1
  In_b/1 -> Logical Operator14/2, Logical Operator16/2, Logical Operator8/2, Logical Operator22/1, Logical Operator4/2, Logical Operator27/1, Logical Operator2/2, Logical Operator12/1
  Logical Operator27/1 -> Logical Operator3/2
  Logical Operator26/1 -> Logical Operator3/1
  Logical Operator25/1 -> Logical Operator2/3
  In_a/1 -> Logical Operator11/1, Logical Operator24/1, Logical Operator14/1, Logical Operator16/1, Logical Operator8/1, Logical Operator7/1, Logical Operator23/1, Logical Operator26/1
  Logical Operator24/1 -> Logical Operator2/1
  Logical Operator23/1 -> Logical Operator4/1
  Logical Operator22/1 -> Logical Operator7/2
  Logical Operator21/1 -> Logical Operator8/3
  Logical Operator20/1 -> Logical Operator17/3
  Logical Operator18/1 -> Logical Operator17/2
  Logical Operator19/1 -> Logical Operator17/1
  Logical Operator14/1 -> Logical Operator15/2
  Logical Operator15/1 -> Logical Operator13/3
  Logical Operator10/1 -> Logical Operator13/2
  Logical Operator9/1 -> Logical Operator13/1
  Logical Operator6/1 -> Logical Operator10/2
  Logical Operator5/1 -> Logical Operator9/2
  Logical Operator8/1 -> Logical Operator6/3
  Logical Operator7/1 -> Logical Operator6/2
  Logical Operator4/1 -> Logical Operator6/1
  Logical Operator3/1 -> Logical Operator5/3
  Logical Operator11/1 -> Logical Operator5/1
  Logical Operator2/1 -> Logical Operator5/2
  Logical Operator1/1 -> Logical Operator11/3
  Logical Operator12/1 -> Logical Operator11/2

== system mylib/264_DZ_trans_st_v1/Poly12_det19_ph/Za/stp_1 ==
  Y_in : Inport
  alg_in : Inport  Port=2
  Re_cur : Inport  Port=3
  Im_cur : Inport  Port=4
  Re_next : Inport  Port=5
  Im_next : Inport  Port=6
  re : Inport  Port=7
  im : Inport  Port=8
  start_pt : Inport  Port=9
  Re_start : Inport  Port=10
  Im_start : Inport  Port=11
  Constant : Constant  Value=0
  Constant1 : Constant  Value=0
  D1 : Logic  AllPortsSameDT=off  OutDataTypeStr=boolean
  Divide : Product  Inputs=**
  Divide1 : Product  Inputs=*/
  Logical Operator1 : Logic  Inputs=3  AllPortsSameDT=off  OutDataTypeStr=boolean
  Logical Operator2 : Logic  AllPortsSameDT=off  OutDataTypeStr=boolean
  Logical Operator3 : Logic  AllPortsSameDT=off  OutDataTypeStr=boolean
  Logical Operator4 : Logic  Operator=OR  AllPortsSameDT=off  OutDataTypeStr=boolean
  Logical Operator5 : Logic  AllPortsSameDT=off  OutDataTypeStr=boolean
  Logical Operator6 : Logic  Operator=OR  AllPortsSameDT=off  OutDataTypeStr=boolean
  Logical Operator7 : Logic  Operator=NOT  AllPortsSameDT=off  OutDataTypeStr=boolean
  Logical Operator8 : Logic  Operator=NOT  AllPortsSameDT=off  OutDataTypeStr=boolean
  Relational Operator{,1..3} (4 alike) : RelationalOperator  Operator===  OutDataTypeStr=boolean  RndMeth=Simplest
  Relational Operator4 : RelationalOperator  Operator=<  OutDataTypeStr=boolean  RndMeth=Simplest
  Relational Operator5 : RelationalOperator  Operator=>  OutDataTypeStr=boolean  RndMeth=Simplest
  Relational Operator6 : RelationalOperator  Operator=<  OutDataTypeStr=boolean  RndMeth=Simplest
  Relational Operator7 : RelationalOperator  Operator=>  OutDataTypeStr=boolean  RndMeth=Simplest
  Relational Operator8 : RelationalOperator  Operator=>  OutDataTypeStr=boolean  RndMeth=Simplest
  Switch{1..6} (6 alike) : Switch  Criteria=u2 > Threshold
  X2-X1 : Sum  Inputs=+-
  Y-Y1 : Sum  Inputs=+-
  Y2-Y1 : Sum  Inputs=+-
  Y2-Y2 : Sum
  Y_out : Outport
  alg_out : Outport  Port=2
  cur_Re : Outport  Port=3
  cur_Im : Outport  Port=4
  wires:
  Constant/1 -> Relational Operator1/2, Relational Operator/2
  Relational Operator1/1 -> D1/1
  Relational Operator/1 -> D1/2
  D1/1 -> Logical Operator1/1, Switch1/2, Switch2/2
  Re_next/1 -> Switch2/3, Relational Operator1/1
  Im_next/1 -> Switch1/3, Relational Operator/1
  Constant1/1 -> Relational Operator3/2, Relational Operator2/2
  Relational Operator2/1 -> Logical Operator1/3
  Relational Operator3/1 -> Logical Operator1/2
  Relational Operator4/1 -> Logical Operator2/1
  Relational Operator5/1 -> Logical Operator2/2
  Relational Operator6/1 -> Logical Operator3/1
  Relational Operator7/1 -> Logical Operator3/2
  Logical Operator2/1 -> Logical Operator4/1
  Logical Operator3/1 -> Logical Operator4/2
  Logical Operator4/1 -> Logical Operator5/1
  Logical Operator1/1 -> Logical Operator7/1
  Logical Operator7/1 -> Logical Operator6/1
  start_pt/1 -> Logical Operator6/2
  X2-X1/1 -> Divide/2
  Divide/1 -> Divide1/1
  Y2-Y1/1 -> Divide1/2
  Y-Y1/1 -> Divide/1
  Divide1/1 -> Y2-Y2/1
  Re_cur/1 -> Relational Operator3/1, X2-X1/2, Switch5/3, Y2-Y2/2
  Im_start/1 -> Switch1/1
  Re_start/1 -> Switch2/1
  re/1 -> Relational Operator8/2
  Y2-Y2/1 -> Relational Operator8/1
  im/1 -> Relational Operator7/1, Relational Operator6/1, Relational Operator5/1, Relational Operator4/1, Y-Y1/1
  Im_cur/1 -> Y2-Y1/2, Y-Y1/2, Relational Operator2/1, Switch6/3, Relational Operator6/2, Relational Operator5/2
  Switch2/1 -> X2-X1/1, Switch5/1
  Switch1/1 -> Y2-Y1/1, Switch6/1, Relational Operator7/2, Relational Operator4/2
  Relational Operator8/1 -> Logical Operator5/2
  Logical Operator5/1 -> Switch3/2
  Logical Operator6/1 -> Switch6/2, Switch5/2, Switch4/2
  Y_in/1 -> Switch4/3
  Switch3/1 -> alg_out/1, Switch4/1
  alg_in/1 -> Logical Operator8/1, Switch3/3
  Logical Operator8/1 -> Switch3/1
  Switch4/1 -> Y_out/1
  Switch6/1 -> cur_Im/1
  Switch5/1 -> cur_Re/1

== system mylib/264_DZ_trans_st_v1/Poly12_det19_ph/Za/stp_10 ==
  Y_in : Inport
  alg_in : Inport  Port=2
  Re_cur : Inport  Port=3
  Im_cur : Inport  Port=4
  Re_next : Inport  Port=5
  Im_next : Inport  Port=6
  re : Inport  Port=7
  im : Inport  Port=8
  start_pt : Inport  Port=9
  Re_start : Inport  Port=10
  Im_start : Inport  Port=11
  Constant : Constant  Value=0
  Constant1 : Constant  Value=0
  D1 : Logic  AllPortsSameDT=off  OutDataTypeStr=boolean
  Divide : Product  Inputs=**
  Divide1 : Product  Inputs=*/
  Logical Operator1 : Logic  Inputs=3  AllPortsSameDT=off  OutDataTypeStr=boolean
  Logical Operator2 : Logic  AllPortsSameDT=off  OutDataTypeStr=boolean
  Logical Operator3 : Logic  AllPortsSameDT=off  OutDataTypeStr=boolean
  Logical Operator4 : Logic  Operator=OR  AllPortsSameDT=off  OutDataTypeStr=boolean
  Logical Operator5 : Logic  AllPortsSameDT=off  OutDataTypeStr=boolean
  Logical Operator6 : Logic  Operator=OR  AllPortsSameDT=off  OutDataTypeStr=boolean
  Logical Operator7 : Logic  Operator=NOT  AllPortsSameDT=off  OutDataTypeStr=boolean
  Logical Operator8 : Logic  Operator=NOT  AllPortsSameDT=off  OutDataTypeStr=boolean
  Relational Operator{,1..3} (4 alike) : RelationalOperator  Operator===  OutDataTypeStr=boolean  RndMeth=Simplest
  Relational Operator4 : RelationalOperator  Operator=<  OutDataTypeStr=boolean  RndMeth=Simplest
  Relational Operator5 : RelationalOperator  Operator=>  OutDataTypeStr=boolean  RndMeth=Simplest
  Relational Operator6 : RelationalOperator  Operator=<  OutDataTypeStr=boolean  RndMeth=Simplest
  Relational Operator7 : RelationalOperator  Operator=>  OutDataTypeStr=boolean  RndMeth=Simplest
  Relational Operator8 : RelationalOperator  Operator=>  OutDataTypeStr=boolean  RndMeth=Simplest
  Switch{1..6} (6 alike) : Switch  Criteria=u2 > Threshold
  X2-X1 : Sum  Inputs=+-
  Y-Y1 : Sum  Inputs=+-
  Y2-Y1 : Sum  Inputs=+-
  Y2-Y2 : Sum
  Y_out : Outport
  alg_out : Outport  Port=2
  cur_Re : Outport  Port=3
  cur_Im : Outport  Port=4
  wires:
  Constant/1 -> Relational Operator1/2, Relational Operator/2
  Relational Operator1/1 -> D1/1
  Relational Operator/1 -> D1/2
  D1/1 -> Logical Operator1/1, Switch1/2, Switch2/2
  Re_next/1 -> Switch2/3, Relational Operator1/1
  Im_next/1 -> Switch1/3, Relational Operator/1
  Constant1/1 -> Relational Operator3/2, Relational Operator2/2
  Relational Operator2/1 -> Logical Operator1/3
  Relational Operator3/1 -> Logical Operator1/2
  Relational Operator4/1 -> Logical Operator2/1
  Relational Operator5/1 -> Logical Operator2/2
  Relational Operator6/1 -> Logical Operator3/1
  Relational Operator7/1 -> Logical Operator3/2
  Logical Operator2/1 -> Logical Operator4/1
  Logical Operator3/1 -> Logical Operator4/2
  Logical Operator4/1 -> Logical Operator5/1
  Logical Operator1/1 -> Logical Operator7/1
  Logical Operator7/1 -> Logical Operator6/1
  start_pt/1 -> Logical Operator6/2
  X2-X1/1 -> Divide/2
  Divide/1 -> Divide1/1
  Y2-Y1/1 -> Divide1/2
  Y-Y1/1 -> Divide/1
  Divide1/1 -> Y2-Y2/1
  Re_cur/1 -> Relational Operator3/1, X2-X1/2, Switch5/3, Y2-Y2/2
  Im_start/1 -> Switch1/1
  Re_start/1 -> Switch2/1
  re/1 -> Relational Operator8/2
  Y2-Y2/1 -> Relational Operator8/1
  im/1 -> Relational Operator7/1, Relational Operator6/1, Relational Operator5/1, Relational Operator4/1, Y-Y1/1
  Im_cur/1 -> Y2-Y1/2, Y-Y1/2, Relational Operator2/1, Switch6/3, Relational Operator6/2, Relational Operator5/2
  Switch2/1 -> X2-X1/1, Switch5/1
  Switch1/1 -> Y2-Y1/1, Switch6/1, Relational Operator7/2, Relational Operator4/2
  Relational Operator8/1 -> Logical Operator5/2
  Logical Operator5/1 -> Switch3/2
  Logical Operator6/1 -> Switch6/2, Switch5/2, Switch4/2
  Y_in/1 -> Switch4/3
  Switch3/1 -> alg_out/1, Switch4/1
  alg_in/1 -> Logical Operator8/1, Switch3/3
  Logical Operator8/1 -> Switch3/1
  Switch4/1 -> Y_out/1
  Switch6/1 -> cur_Im/1
  Switch5/1 -> cur_Re/1

== system mylib/264_DZ_trans_st_v1/Poly12_det19_ph/Za/stp_11 ==
  Y_in : Inport
  alg_in : Inport  Port=2
  Re_cur : Inport  Port=3
  Im_cur : Inport  Port=4
  Re_next : Inport  Port=5
  Im_next : Inport  Port=6
  re : Inport  Port=7
  im : Inport  Port=8
  start_pt : Inport  Port=9
  Re_start : Inport  Port=10
  Im_start : Inport  Port=11
  Constant : Constant  Value=0
  Constant1 : Constant  Value=0
  D1 : Logic  AllPortsSameDT=off  OutDataTypeStr=boolean
  Divide : Product  Inputs=**
  Divide1 : Product  Inputs=*/
  Logical Operator1 : Logic  Inputs=3  AllPortsSameDT=off  OutDataTypeStr=boolean
  Logical Operator2 : Logic  AllPortsSameDT=off  OutDataTypeStr=boolean
  Logical Operator3 : Logic  AllPortsSameDT=off  OutDataTypeStr=boolean
  Logical Operator4 : Logic  Operator=OR  AllPortsSameDT=off  OutDataTypeStr=boolean
  Logical Operator5 : Logic  AllPortsSameDT=off  OutDataTypeStr=boolean
  Logical Operator6 : Logic  Operator=OR  AllPortsSameDT=off  OutDataTypeStr=boolean
  Logical Operator7 : Logic  Operator=NOT  AllPortsSameDT=off  OutDataTypeStr=boolean
  Logical Operator8 : Logic  Operator=NOT  AllPortsSameDT=off  OutDataTypeStr=boolean
  Relational Operator{,1..3} (4 alike) : RelationalOperator  Operator===  OutDataTypeStr=boolean  RndMeth=Simplest
  Relational Operator4 : RelationalOperator  Operator=<  OutDataTypeStr=boolean  RndMeth=Simplest
  Relational Operator5 : RelationalOperator  Operator=>  OutDataTypeStr=boolean  RndMeth=Simplest
  Relational Operator6 : RelationalOperator  Operator=<  OutDataTypeStr=boolean  RndMeth=Simplest
  Relational Operator7 : RelationalOperator  Operator=>  OutDataTypeStr=boolean  RndMeth=Simplest
  Relational Operator8 : RelationalOperator  Operator=>  OutDataTypeStr=boolean  RndMeth=Simplest
  Switch{1..6} (6 alike) : Switch  Criteria=u2 > Threshold
  X2-X1 : Sum  Inputs=+-
  Y-Y1 : Sum  Inputs=+-
  Y2-Y1 : Sum  Inputs=+-
  Y2-Y2 : Sum
  Y_out : Outport
  alg_out : Outport  Port=2
  cur_Re : Outport  Port=3
  cur_Im : Outport  Port=4
  wires:
  Constant/1 -> Relational Operator1/2, Relational Operator/2
  Relational Operator1/1 -> D1/1
  Relational Operator/1 -> D1/2
  D1/1 -> Logical Operator1/1, Switch1/2, Switch2/2
  Re_next/1 -> Switch2/3, Relational Operator1/1
  Im_next/1 -> Switch1/3, Relational Operator/1
  Constant1/1 -> Relational Operator3/2, Relational Operator2/2
  Relational Operator2/1 -> Logical Operator1/3
  Relational Operator3/1 -> Logical Operator1/2
  Relational Operator4/1 -> Logical Operator2/1
  Relational Operator5/1 -> Logical Operator2/2
  Relational Operator6/1 -> Logical Operator3/1
  Relational Operator7/1 -> Logical Operator3/2
  Logical Operator2/1 -> Logical Operator4/1
  Logical Operator3/1 -> Logical Operator4/2
  Logical Operator4/1 -> Logical Operator5/1
  Logical Operator1/1 -> Logical Operator7/1
  Logical Operator7/1 -> Logical Operator6/1
  start_pt/1 -> Logical Operator6/2
  X2-X1/1 -> Divide/2
  Divide/1 -> Divide1/1
  Y2-Y1/1 -> Divide1/2
  Y-Y1/1 -> Divide/1
  Divide1/1 -> Y2-Y2/1
  Re_cur/1 -> Relational Operator3/1, X2-X1/2, Switch5/3, Y2-Y2/2
  Im_start/1 -> Switch1/1
  Re_start/1 -> Switch2/1
  re/1 -> Relational Operator8/2
  Y2-Y2/1 -> Relational Operator8/1
  im/1 -> Relational Operator7/1, Relational Operator6/1, Relational Operator5/1, Relational Operator4/1, Y-Y1/1
  Im_cur/1 -> Y2-Y1/2, Y-Y1/2, Relational Operator2/1, Switch6/3, Relational Operator6/2, Relational Operator5/2
  Switch2/1 -> X2-X1/1, Switch5/1
  Switch1/1 -> Y2-Y1/1, Switch6/1, Relational Operator7/2, Relational Operator4/2
  Relational Operator8/1 -> Logical Operator5/2
  Logical Operator5/1 -> Switch3/2
  Logical Operator6/1 -> Switch6/2, Switch5/2, Switch4/2
  Y_in/1 -> Switch4/3
  Switch3/1 -> alg_out/1, Switch4/1
  alg_in/1 -> Logical Operator8/1, Switch3/3
  Logical Operator8/1 -> Switch3/1
  Switch4/1 -> Y_out/1
  Switch6/1 -> cur_Im/1
  Switch5/1 -> cur_Re/1
